simulink model "prob_5"  (R2020b)
settings: Solver=VariableStepAuto  StartTime=0.0  StopTime=10.0  FixedStep=0.001  MaxStep=0.001  RelTol=1e-3
values from neighbouring files (symbols this model uses):
  C = 10^-5    (= 1e-05)    [Initializing_prob5.m]
  R = 10    [Initializing_prob5.m]
settings Model: Creator=Lakshmi  LastModifiedBy=Lakshmi

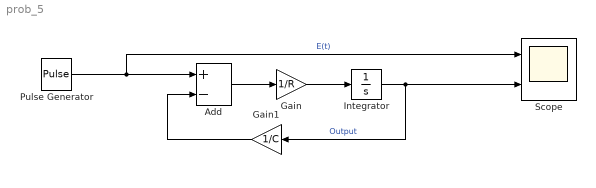
== system prob_5 ==
  Add : Sum  Inputs=+-
  Gain : Gain  Gain=1/R
  Gain1 : Gain  Gain=1/C
  Integrator : Integrator  InitialCondition=10
  Pulse Generator : DiscretePulseGenerator  PulseType=Time based  Period=5  PulseWidth=5
  Scope : Scope  NumInputPorts=2
  wires:
  Integrator/1 -> Scope/2, Gain1/1  "Output"
  Gain/1 -> Integrator/1
  Add/1 -> Gain/1
  Pulse Generator/1 -> Scope/1, Add/1  "E(t)"
  Gain1/1 -> Add/2
